simulink model "major"  (Simulink 7.4)
settings: Solver=ode23tb  StartTime=0.0  StopTime=2.5  RelTol=1e-3
InitFcn:
  | Ts=20e-6;
undefined symbols (not defined in the file): DiscIntNeverNeededParam, fc
libraries: powerlib x97, simulink x12, powerlib_extras x2
settings Model: Creator=srikanth  LastModifiedBy=Anil Pavuluru
settings DataIOCC: SaveOutput=off  SaveTime=off
settings DebuggingCC: AlgebraicLoopMsg=none

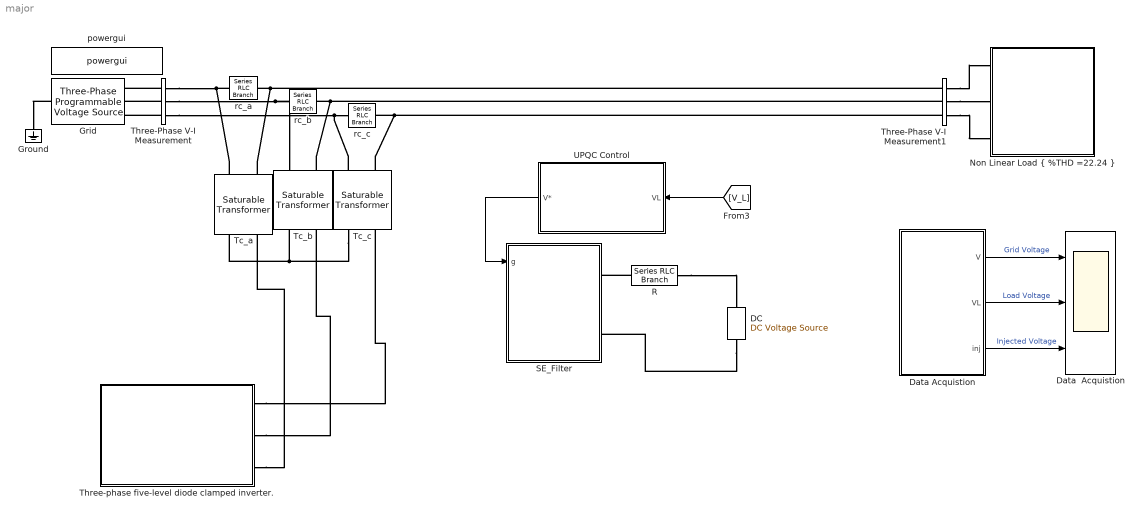
== system major ==
  DC : powerlib/Electrical Sources/DC Voltage Source  DialogController=POWERSYS.PowerSysDialog  SystemSampleTime=-1  Amplitude=700  Measurements=None
  Data  Acquistion : Scope  NumInputPorts=3
      settings: TickLabels=on  TimeRange=2.5  YMin=-350~-300~-200  YMax=350~350~225  SaveName=se_pi1
  Data Acquistion : Subsystem
      mask Display: fprintf('scopes')
  Grid : powerlib/Electrical Sources/Three-Phase Programmable Voltage Source  DialogController=POWERSYS.PowerSysDialog  SystemSampleTime=-1  PositiveSequence="[380  0 50]"  VariationEntity=Amplitude  VariationType=Table of time-amplitude pairs  VariationStep=0.5  VariationRate=10  VariationMagnitude=0.3  VariationFrequency=2  VariationTiming=[1 2]  VariationPhaseA=off  Amplitudes=[1 0.5 1 1.5 1]  TimeValues=[0 0.5 0.7 1.5 1.7]  HarmonicGeneration=on  HarmonicA=[5 0.2 0 2]  HarmonicB=[7 0.05 0 1]  Timing="[0.2  0.4]"
  Ground : powerlib/Elements/Ground  DialogController=POWERSYS.PowerSysDialog  PhysicalDomain=powersysdomain  SubClassName=unknown  LeftPortType=p1  RightPortType=p1  LConnTagsString=a
  "Non Linear Load { %THD =22.24 }" : Subsystem
      mask Display: fprintf('Non Linear\nLoad')
  R : powerlib/Elements/Series RLC Branch  DialogController=POWERSYS.PowerSysDialog  PhysicalDomain=powersysdomain  SubClassName=unknown  LeftPortType=p1  RightPortType=p1  LConnTagsString=__new0  RConnTagsString=__new0  BranchType=R  Resistance=0.1  Inductance=1e-3  SetiL0=off  InitialCurrent=0  Capacitance=1e-6  Setx0=off  InitialVoltage=0  Measurements=None
  SE_Filter : Subsystem
      mask Display: fprintf('series\nfilter')
  Tc_a : powerlib/Elements/Saturable Transformer  DialogController=POWERSYS.PowerSysDialog  SystemSampleTime=-1  ThreeWindings=off  UNITS=pu  NominalPower=[4000 50]  Winding1="[380  0.02  0.02 ]"  Winding2="[380  0.02  0.02]"  Winding3="[ 315e3  0.002  0.08 ]"  Saturation=[ 0 0 ;1.016 9.043]*1e-3  CoreLoss=[117 0]  Hysteresis=off  DataFile='hysteresis.mat'  Measurements=None  MoreParameters=off  BreakLoop=off  DataType=off  InitialFlux=0  TransfoNumber=1
  Tc_b : powerlib/Elements/Saturable Transformer  DialogController=POWERSYS.PowerSysDialog  SystemSampleTime=-1  ThreeWindings=off  UNITS=pu  NominalPower=[4000 50]  Winding1="[380  0.02  0.02 ]"  Winding2="[380  0.02  0.02]"  Winding3="[ 315e3  0.002  0.08 ]"  Saturation=[ 0 0 ;1.016 9.043]*1e-3  CoreLoss=[117 0]  Hysteresis=off  DataFile='hysteresis.mat'  Measurements=None  MoreParameters=off  BreakLoop=off  DataType=off  InitialFlux=0  TransfoNumber=1
  Tc_c : powerlib/Elements/Saturable Transformer  DialogController=POWERSYS.PowerSysDialog  SystemSampleTime=-1  ThreeWindings=off  UNITS=pu  NominalPower=[4000 50]  Winding1="[380  0.02  0.02 ]"  Winding2="[380  0.02  0.02]"  Winding3="[ 315e3  0.002  0.08 ]"  Saturation=[ 0 0 ;1.016 9.043]*1e-3  CoreLoss=[117 0]  Hysteresis=off  DataFile='hysteresis.mat'  Measurements=None  MoreParameters=off  BreakLoop=off  DataType=off  InitialFlux=0  TransfoNumber=1
  Three-Phase V-I Measurement : powerlib/Measurements/Three-Phase V-I Measurement  DialogController=POWERSYS.PowerSysDialog  SystemSampleTime=-1  VoltageMeasurement=phase-to-ground  SetLabelV=on  LabelV=Vabc  Vpu=off  CurrentMeasurement=yes  SetLabelI=on  LabelI=Iabc  Ipu=off  Pbase=100e6  Vbase=500e3  OutputType=Complex  PhasorSimulation=off  PSBequivalent=0
  Three-Phase V-I Measurement1 : powerlib/Measurements/Three-Phase V-I Measurement  DialogController=POWERSYS.PowerSysDialog  SystemSampleTime=-1  VoltageMeasurement=phase-to-ground  SetLabelV=on  LabelV=V_L  Vpu=off  CurrentMeasurement=yes  SetLabelI=on  LabelI=I_L  Ipu=off  Pbase=100e6  Vbase=500e3  OutputType=Complex  PhasorSimulation=off  PSBequivalent=0
  Three-phase five-level diode clamped inverter. : Subsystem
  UPQC Control : Subsystem
      mask Display: fprintf('Series\nFilter')
  powergui : powerlib/powergui  Priority=1  SystemSampleTime=-1  SimulationMode=Discrete  SampleTime=Ts  frequency=60  SPID=off  DisableSnubberDevices=off  DisableRonSwitches=off  DisableVfSwitches=off  SwTol=0  Interpol=off  frequencyindice=50  echomessages=off  HookPort=off  DisplayEquations=off  FunctionMessages=off  EnableUseOfTLC=off  x0status=blocks  RestoreLinks=warning  Frange=[0:2:500]  Ylog=off  Xlog=on  ShowGrid=off  save=off  variable=ZData  structure=voltage_pi  ZoomFFT=off  StartTime=1.5  cycles=10  DisplayStyle=1  fundamental=50  FreqAxis=on  MaxFrequency=1000  frequencyindicesteady=1  RmsSteady=1  display=off  Ts=0  methode=off
  rc_a : powerlib/Elements/Series RLC Branch  DialogController=POWERSYS.PowerSysDialog  PhysicalDomain=powersysdomain  SubClassName=unknown  LeftPortType=p1  RightPortType=p1  LConnTagsString=__new0  RConnTagsString=__new0  BranchType=RC  Resistance=1  Inductance=1e-3  SetiL0=off  InitialCurrent=0  Capacitance=100e-6  Setx0=off  InitialVoltage=0  Measurements=Branch voltage
  rc_b : powerlib/Elements/Series RLC Branch  DialogController=POWERSYS.PowerSysDialog  PhysicalDomain=powersysdomain  SubClassName=unknown  LeftPortType=p1  RightPortType=p1  LConnTagsString=__new0  RConnTagsString=__new0  BranchType=RC  Resistance=1  Inductance=1e-3  SetiL0=off  InitialCurrent=0  Capacitance=100e-6  Setx0=off  InitialVoltage=0  Measurements=Branch voltage
  rc_c : powerlib/Elements/Series RLC Branch  DialogController=POWERSYS.PowerSysDialog  PhysicalDomain=powersysdomain  SubClassName=unknown  LeftPortType=p1  RightPortType=p1  LConnTagsString=__new0  RConnTagsString=__new0  BranchType=RC  Resistance=1  Inductance=1e-3  SetiL0=off  InitialCurrent=0  Capacitance=100e-6  Setx0=off  InitialVoltage=0  Measurements=Branch voltage
  wires:
  [V_L] -> UPQC Control/1(VL)
  UPQC Control/1(V*) -> SE_Filter/1(g)
  Data Acquistion/1(V) -> Data  Acquistion/1  "Grid Voltage"
  Data Acquistion/2(VL) -> Data  Acquistion/2  "Load Voltage"
  Data Acquistion/3("inj ") -> Data  Acquistion/3  "Injected Voltage"
  connections:
  Three-Phase V-I Measurement1/LConn2 -- rc_b/LConn1 -- Tc_b/RConn2
  Three-Phase V-I Measurement1/LConn1 -- rc_a/LConn1 -- Tc_a/RConn2
  Grid/LConn1 -- Ground/LConn1
  Three-Phase V-I Measurement/LConn1 -- Grid/RConn1
  Three-Phase V-I Measurement/LConn2 -- Grid/RConn2
  Three-Phase V-I Measurement/LConn3 -- Grid/RConn3
  Three-Phase V-I Measurement1/RConn2 -- "Non Linear Load { %THD =22.24 }"/LConn2
  Three-Phase V-I Measurement1/LConn3 -- rc_c/LConn1 -- Tc_c/RConn2
  rc_a/RConn1 -- Three-Phase V-I Measurement/RConn1 -- Tc_a/RConn1
  rc_b/RConn1 -- Three-Phase V-I Measurement/RConn2 -- Tc_b/RConn1
  rc_c/RConn1 -- Three-Phase V-I Measurement/RConn3 -- Tc_c/RConn1
  Three-Phase V-I Measurement1/RConn3 -- "Non Linear Load { %THD =22.24 }"/LConn3
  Three-Phase V-I Measurement1/RConn1 -- "Non Linear Load { %THD =22.24 }"/LConn1
  Three-phase five-level diode clamped inverter./RConn3 -- Tc_a/LConn2
  Three-phase five-level diode clamped inverter./RConn2 -- Tc_b/LConn2
  Three-phase five-level diode clamped inverter./RConn1 -- Tc_c/LConn2
  Tc_c/LConn1 -- Tc_a/LConn1 -- Tc_b/LConn1
  R/LConn1 -- SE_Filter/RConn1
  R/RConn1 -- DC/RConn1
  DC/LConn1 -- SE_Filter/RConn2

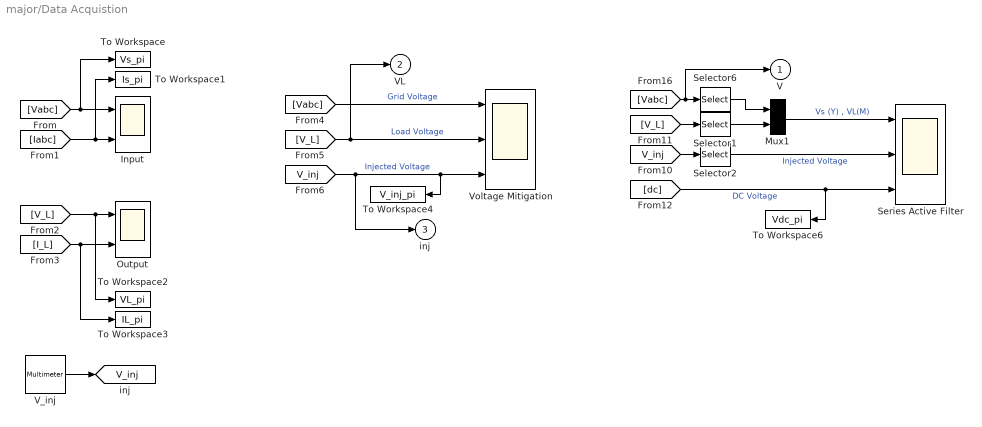
== system major/Data Acquistion ==
  Input : Scope  NumInputPorts=2
      settings: TimeRange=0.1  YMin=-400~-15  YMax=400~15  SaveName=Grid_pi
  Mux1 : Mux  Inputs=2
      settings: DisplayOption=signals
  Output : Scope  NumInputPorts=2
      settings: TimeRange=0.1  YMin=-400~-10  YMax=400~10  SaveName=Load_pi
  Selector1 : Selector  InputPortWidth=3  IndexOptions=Index vector (dialog)  Indices=1  OutputSizes=1
  Selector2 : Selector  InputPortWidth=3  IndexOptions=Index vector (dialog)  Indices=1  OutputSizes=1
  Selector6 : Selector  InputPortWidth=3  IndexOptions=Index vector (dialog)  Indices=1  OutputSizes=1
  Series Active Filter : Scope  NumInputPorts=3
      settings: TickLabels=on  TimeRange=2  YMin=-350~-175~600  YMax=350~175~1000  SaveName=se_pi
  To Workspace : ToWorkspace  VariableName=Vs_pi  SampleTime=Ts  SaveFormat=Array
  To Workspace1 : ToWorkspace  VariableName=Is_pi  SampleTime=Ts  SaveFormat=Array
  To Workspace2 : ToWorkspace  VariableName=VL_pi  SampleTime=Ts  SaveFormat=Array
  To Workspace3 : ToWorkspace  VariableName=IL_pi  SampleTime=Ts  SaveFormat=Array
  To Workspace4 : ToWorkspace  VariableName=V_inj_pi  SampleTime=Ts  SaveFormat=Array
  To Workspace6 : ToWorkspace  VariableName=Vdc_pi  SampleTime=Ts  SaveFormat=Array
  V_inj : powerlib/Measurements/Multimeter  SystemSampleTime=-1  PhasorSimulation=off  OutputType=Complex  sel=[1 2 3]  L=7  Gain=[1 1 1]  yselected={'Ub: rc_a','Ub: rc_b','Ub: rc_c'};  PSBOutputType=1  PSBequivalent=0  AxesSetting=[0,0.1,-100,100]  Display=0  SavedBlockNames=-11
  Voltage Mitigation : Scope  NumInputPorts=3
      settings: TimeRange=0.2  YMin=-500~-500~-200  YMax=500~500~200  SaveName=voltage_pi
  V : Outport  OutDataType=fixdt(1, 16)  OutScaling=2^0
  VL : Outport  Port=2  OutDataType=fixdt(1, 16)  OutScaling=2^0
  "inj " : Outport  Port=3  OutDataType=fixdt(1, 16)  OutScaling=2^0
  tag scope: V_inj=global
  wires:
  [Vabc] -> Input/1, To Workspace/1
  [Iabc] -> Input/2, To Workspace1/1
  [V_L] -> Output/1, To Workspace2/1
  [I_L] -> Output/2, To Workspace3/1
  [Vabc] -> Voltage Mitigation/1  "Grid Voltage"
  [V_L] -> Voltage Mitigation/2, VL/1  "Load Voltage"
  [V_inj] -> Voltage Mitigation/3, To Workspace4/1, "inj "/1  "Injected Voltage"
  [V_L] -> Selector1/1
  [V_inj] -> Selector2/1
  [dc] -> Series Active Filter/3, To Workspace6/1  "DC Voltage"
  Selector2/1 -> Series Active Filter/2  "Injected Voltage"
  [Vabc] -> Selector6/1, V/1
  Selector1/1 -> Mux1/2
  Mux1/1 -> Series Active Filter/1  "Vs (Y) , VL(M)"
  Selector6/1 -> Mux1/1
  V_inj/1 -> [V_inj]

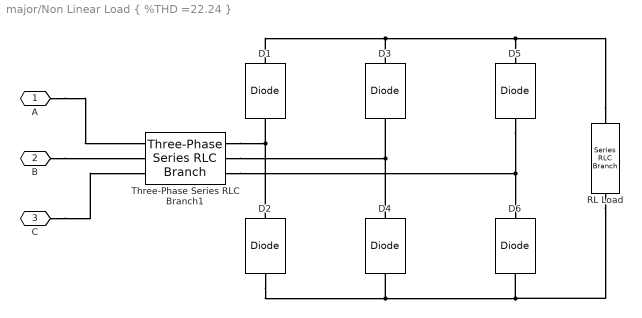
== system major/Non Linear Load { %THD =22.24 } ==
  D{1..6} (6 alike) : powerlib/Power Electronics/Diode  DialogController=POWERSYS.PowerSysDialog  SystemSampleTime=-1  Ron=0.001  Lon=0  Vf=0.8  IC=0  UseSnubber=off  Rs=500  Cs=250e-9  Measurements=off
  RL Load : powerlib/Elements/Series RLC Branch  DialogController=POWERSYS.PowerSysDialog  PhysicalDomain=powersysdomain  SubClassName=unknown  LeftPortType=p1  RightPortType=p1  LConnTagsString=__new0  RConnTagsString=__new0  BranchType=RL  Resistance=60  Inductance=0.15e-3  SetiL0=off  InitialCurrent=0  Capacitance=1e-6  Setx0=off  InitialVoltage=0  Measurements=None
  Three-Phase Series RLC Branch1 : powerlib/Elements/Three-Phase Series RLC Branch  DialogController=POWERSYS.PowerSysDialog  PhysicalDomain=powersysdomain  SubClassName=unknown  LeftPortType=p1  RightPortType=p1  LConnTagsString=A|B|C  RConnTagsString=A|B|C  BranchType=RL  Resistance=0.4  Inductance=15e-3  Capacitance=1e-6  Measurements=None
  A : PMIOPort  Port=1  Side=Left
  B : PMIOPort  Port=2  Side=Left
  C : PMIOPort  Port=3  Side=Left
  connections:
  C/RConn1 -- Three-Phase Series RLC Branch1/LConn3
  B/RConn1 -- Three-Phase Series RLC Branch1/LConn2
  A/RConn1 -- Three-Phase Series RLC Branch1/LConn1
  Three-Phase Series RLC Branch1/RConn3 -- D6/RConn1 -- D5/LConn1
  Three-Phase Series RLC Branch1/RConn2 -- D4/RConn1 -- D3/LConn1
  RL Load/RConn1 -- D6/LConn1 -- D4/LConn1 -- D2/LConn1
  RL Load/LConn1 -- D5/RConn1 -- D3/RConn1 -- D1/RConn1
  Three-Phase Series RLC Branch1/RConn1 -- D2/RConn1 -- D1/LConn1

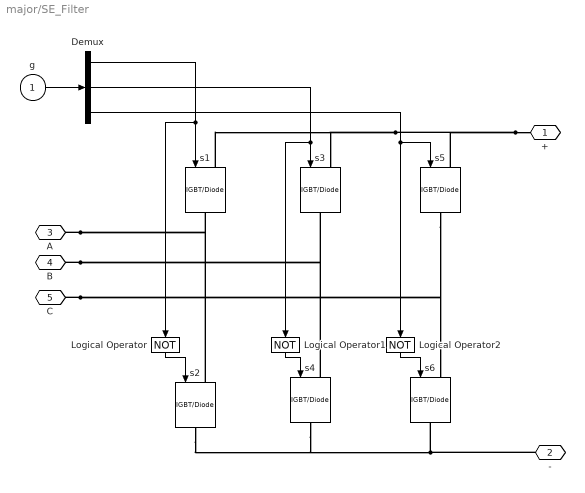
== system major/SE_Filter ==
  g : Inport
  Demux : Demux  Outputs=3
  Logical Operator : Logic  Operator=NOT  AllPortsSameDT=off  OutDataTypeMode=boolean  LogicDataType=fixdt(0, 8)  OutDataTypeStr=boolean
  Logical Operator1 : Logic  Operator=NOT  AllPortsSameDT=off  OutDataTypeMode=boolean  LogicDataType=fixdt(0, 8)  OutDataTypeStr=boolean
  Logical Operator2 : Logic  Operator=NOT  AllPortsSameDT=off  OutDataTypeMode=boolean  LogicDataType=fixdt(0, 8)  OutDataTypeStr=boolean
  s{1..6} (6 alike) : powerlib/Power Electronics/IGBT//Diode  DialogController=POWERSYS.PowerSysDialog  SystemSampleTime=-1  Ron=1e-3  Rs=1e5  Cs=inf  Measurements=off
  + : PMIOPort  Port=1  Side=Right
  - : PMIOPort  Port=2  Side=Right
  A : PMIOPort  Port=3  Side=Left
  B : PMIOPort  Port=4  Side=Left
  C : PMIOPort  Port=5  Side=Left
  wires:
  Demux/2 -> s3/1, Logical Operator1/1
  Demux/1 -> s1/1, Logical Operator/1
  Logical Operator/1 -> s2/1
  Logical Operator1/1 -> s4/1
  Logical Operator2/1 -> s6/1
  Demux/3 -> Logical Operator2/1, s5/1
  g/1 -> Demux/1
  connections:
  +/RConn1 -- s5/LConn1 -- s1/LConn1 -- s3/LConn1
  A/RConn1 -- s2/LConn1 -- s1/RConn1
  -/RConn1 -- s6/RConn1 -- s4/RConn1 -- s2/RConn1
  B/RConn1 -- s4/LConn1 -- s3/RConn1
  C/RConn1 -- s5/RConn1 -- s6/LConn1

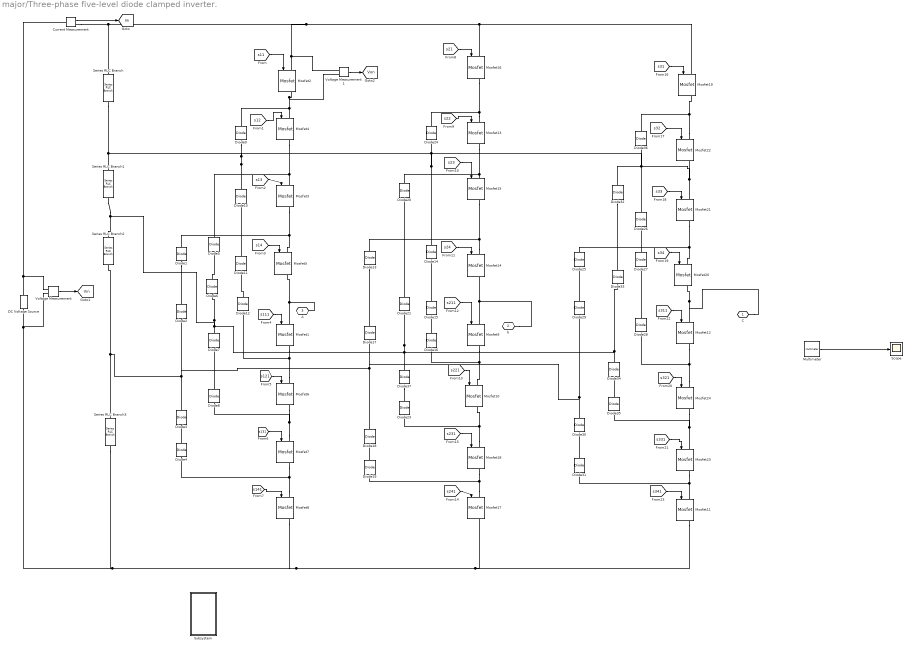
== system major/Three-phase five-level diode clamped inverter. ==
  Current Measurement : powerlib/Measurements/Current Measurement  DialogController=POWERSYS.PowerSysDialog  SystemSampleTime=-1  PhasorSimulation=off  OutputType=Complex  PSBequivalent=0
  DC Voltage Source : powerlib/Electrical Sources/DC Voltage Source  DialogController=POWERSYS.PowerSysDialog  SystemSampleTime=-1  Amplitude=500  Measurements=None
  Diode{1..21,23..37} (36 alike) : powerlib/Power Electronics/Diode  DialogController=POWERSYS.PowerSysDialog  SystemSampleTime=-1  Ron=0.001  Lon=0  Vf=0.8  IC=0  UseSnubber=off  Rs=500  Cs=250e-9  Measurements=off
  Mosfet{1..24} (24 alike) : powerlib/Power Electronics/Mosfet  DialogController=POWERSYS.PowerSysDialog  SystemSampleTime=-1  Ron=0.1  Lon=0  Rd=0.01  Vfd=0  IC=0  Rs=1e5  Cs=inf  Measurements=on
  Multimeter : powerlib/Measurements/Multimeter  SystemSampleTime=-1  PhasorSimulation=off  OutputType=Complex  sel=[4 5 6 7]  L=7  Gain=[1 1 1 1]  yselected={'Ub: Three-phase five-level diode clamped inverter./Series RLC Branch','Ub: Three-phase five-level diode clamped inverter./Series RLC Branch1','Ub: Three-phase five-level diode clamped inverter./Series RLC Branch2','Ub: Three-phase five-level diode clamped inverter./Series RLC Branch3'};  PSBOutputType=1  PSBequivalent=0  AxesSetting=[0,0.1,-100,100]  Display=0  SavedBlockNames=-11
  Scope : Scope
      settings: YMin=-150  YMax=150  SaveName=ScopeData4
  Series RLC Branch{,1..3} (4 alike) : powerlib/Elements/Series RLC Branch  DialogController=POWERSYS.PowerSysDialog  PhysicalDomain=powersysdomain  SubClassName=unknown  LeftPortType=p1  RightPortType=p1  LConnTagsString=__new0  RConnTagsString=__new0  BranchType=RC  Resistance=0.01  Inductance=1e-3  SetiL0=off  InitialCurrent=0  Capacitance=200e-3  Setx0=off  InitialVoltage=0  Measurements=Branch voltage
  Subsystem : Subsystem
  Voltage Measurement : powerlib/Measurements/Voltage Measurement  DialogController=POWERSYS.PowerSysDialog  SystemSampleTime=-1  PhasorSimulation=off  OutputType=Complex  PSBequivalent=0
  Voltage Measurement1 : powerlib/Measurements/Voltage Measurement  DialogController=POWERSYS.PowerSysDialog  SystemSampleTime=-1  PhasorSimulation=off  OutputType=Complex  PSBequivalent=0
  C : PMIOPort  Tag=PMCPort  Port=1  Side=Right
  b : PMIOPort  Tag=PMCPort  Port=2  Side=Right
  A : PMIOPort  Tag=PMCPort  Port=3  Side=Right
  tag scope: Iin=global, Vin=global, Von=global
  wires:
  [s141] -> Mosfet8/1
  [s131] -> Mosfet7/1
  [s121] -> Mosfet6/1
  [s111] -> Mosfet1/1
  [s14] -> Mosfet5/1
  [s13] -> Mosfet3/1
  [s12] -> Mosfet4/1
  [s11] -> Mosfet2/1
  [s241] -> Mosfet17/1
  [s231] -> Mosfet18/1
  [s221] -> Mosfet10/1
  [s211] -> Mosfet9/1
  [s24] -> Mosfet14/1
  [s23] -> Mosfet15/1
  [s22] -> Mosfet13/1
  [s21] -> Mosfet16/1
  [s341] -> Mosfet11/1
  [s331] -> Mosfet23/1
  [s321] -> Mosfet24/1
  [s311] -> Mosfet12/1
  [s34] -> Mosfet20/1
  [s33] -> Mosfet21/1
  [s32] -> Mosfet22/1
  [s31] -> Mosfet19/1
  Multimeter/1 -> Scope/1
  Current Measurement/1 -> [Iin]
  Voltage Measurement/1 -> [Vin]
  Voltage Measurement1/1 -> [Von]
  connections:
  Series RLC Branch3/LConn1 -- Mosfet17/RConn1 -- Mosfet11/RConn1 -- Mosfet8/RConn1 -- DC Voltage Source/LConn1 -- Voltage Measurement/LConn2
  Mosfet16/LConn1 -- Mosfet19/LConn1 -- Series RLC Branch/LConn1 -- Current Measurement/RConn1 -- Mosfet2/LConn1 -- Voltage Measurement1/LConn1
  Series RLC Branch3/RConn1 -- Diode3/RConn1 -- Diode2/LConn1 -- Diode18/RConn1 -- Diode17/LConn1 -- Diode30/RConn1 -- Diode29/LConn1 -- Series RLC Branch2/LConn1
  Mosfet5/LConn1 -- Diode1/RConn1 -- Mosfet3/RConn1
  Diode11/RConn1 -- Diode10/LConn1
  Series RLC Branch1/LConn1 -- Diode10/RConn1 -- Diode9/LConn1 -- Diode14/RConn1 -- Diode24/LConn1 -- Diode26/RConn1 -- Diode36/LConn1 -- Series RLC Branch/RConn1
  Diode12/RConn1 -- Diode11/LConn1
  Mosfet6/LConn1 -- Diode12/LConn1 -- Mosfet1/RConn1
  Mosfet14/LConn1 -- Diode13/RConn1 -- Mosfet15/RConn1
  Diode15/RConn1 -- Diode14/LConn1
  Diode16/RConn1 -- Diode15/LConn1
  Mosfet10/LConn1 -- Diode16/LConn1 -- Mosfet9/RConn1
  Diode19/RConn1 -- Diode18/LConn1
  Mosfet17/LConn1 -- Diode19/LConn1 -- Mosfet18/RConn1
  Diode21/RConn1 -- Diode20/LConn1
  Diode37/LConn1 -- Diode23/RConn1
  Mosfet18/LConn1 -- Diode23/LConn1 -- Mosfet10/RConn1
  Mosfet13/LConn1 -- Diode24/RConn1 -- Mosfet16/RConn1
  Mosfet20/LConn1 -- Diode25/RConn1 -- Mosfet21/RConn1
  Diode27/RConn1 -- Diode26/LConn1
  Diode28/RConn1 -- Diode27/LConn1
  Mosfet24/LConn1 -- Diode28/LConn1 -- Mosfet12/RConn1
  Diode4/RConn1 -- Diode3/LConn1
  Diode31/RConn1 -- Diode30/LConn1
  Mosfet23/RConn1 -- Diode31/LConn1 -- Mosfet11/LConn1
  Mosfet21/LConn1 -- Diode32/RConn1 -- Mosfet22/RConn1
  Series RLC Branch2/RConn1 -- Diode34/RConn1 -- Diode33/LConn1 -- Diode37/RConn1 -- Diode21/LConn1 -- Diode7/RConn1 -- Diode6/LConn1 -- Series RLC Branch1/RConn1
  Diode35/RConn1 -- Diode34/LConn1
  Mosfet24/RConn1 -- Diode35/LConn1 -- Mosfet23/LConn1
  Mosfet22/LConn1 -- Diode36/RConn1 -- Mosfet19/RConn1
  Mosfet8/LConn1 -- Diode4/LConn1 -- Mosfet7/RConn1
  Diode6/RConn1 -- Diode5/LConn1
  Diode8/RConn1 -- Diode7/LConn1
  Mosfet7/LConn1 -- Diode8/LConn1 -- Mosfet6/RConn1
  Mosfet2/RConn1 -- Mosfet4/LConn1 -- Diode9/RConn1 -- Voltage Measurement1/LConn2
  Mosfet9/LConn1 -- b/RConn1 -- Mosfet14/RConn1
  Mosfet1/LConn1 -- A/RConn1 -- Mosfet5/RConn1
  Mosfet12/LConn1 -- C/RConn1 -- Mosfet20/RConn1
  Diode29/RConn1 -- Diode25/LConn1
  Diode1/LConn1 -- Diode2/RConn1
  Diode32/LConn1 -- Diode33/RConn1
  Diode5/RConn1 -- Mosfet3/LConn1 -- Mosfet4/RConn1
  Mosfet13/RConn1 -- Mosfet15/LConn1 -- Diode20/RConn1
  Diode13/LConn1 -- Diode17/RConn1
  DC Voltage Source/RConn1 -- Current Measurement/LConn1 -- Voltage Measurement/LConn1

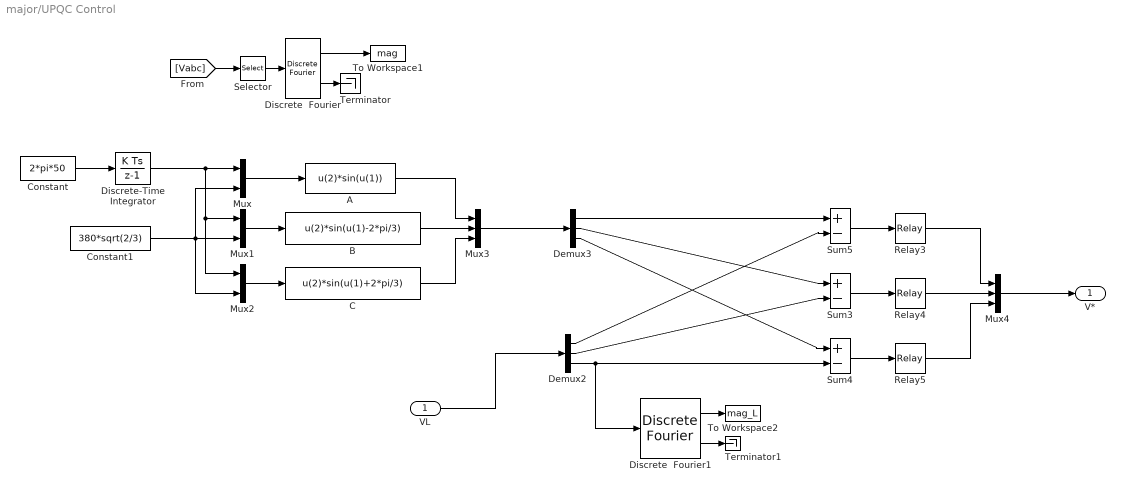
== system major/UPQC Control ==
  VL : Inport
  A : Fcn  Expr=u(2)*sin(u(1))
  B : Fcn  Expr=u(2)*sin(u(1)-2*pi/3)
  C : Fcn  Expr=u(2)*sin(u(1)+2*pi/3)
  Constant : Constant  Value=2*pi*50  OutDataType=fixdt(1, 16)  OutScaling=2^0
  Constant1 : Constant  Value=380*sqrt(2/3)  OutDataType=fixdt(1, 16)  OutScaling=2^0
  Demux2 : Demux  Outputs=3
  Demux3 : Demux  Outputs=3
  Discrete  Fourier : powerlib_extras/Discrete Measurements/Discrete  Fourier  DialogController=POWERSYS.PowerSysDialog  SystemSampleTime=-1  Freq=50  n=1  Par_Init=[0 0]  Ts=Ts
  Discrete  Fourier1 : powerlib_extras/Discrete Measurements/Discrete  Fourier  DialogController=POWERSYS.PowerSysDialog  SystemSampleTime=-1  Freq=50  n=1  Par_Init=[0 0]  Ts=Ts
  Discrete-Time Integrator : DiscreteIntegrator  SampleTime=Ts  OutDataType=fixdt(1, 16)  OutScaling=2^0  ICPrevOutput=DiscIntNeverNeededParam  ICPrevScaledInput=DiscIntNeverNeededParam
  Mux : Mux  Inputs=2
  Mux1 : Mux  Inputs=2
  Mux2 : Mux  Inputs=2
  Mux3 : Mux  Inputs=3
  Mux4 : Mux  Inputs=3
  Relay3 : Relay  OnSwitchValue=1  OffSwitchValue=-1  OutDataType=fixdt(1, 16)  OutScaling=2^0
  Relay4 : Relay  OnSwitchValue=1  OffSwitchValue=-1  OutDataType=fixdt(1, 16)  OutScaling=2^0
  Relay5 : Relay  OnSwitchValue=1  OffSwitchValue=-1  OutDataType=fixdt(1, 16)  OutScaling=2^0
  Selector : Selector  InputPortWidth=3  IndexOptions=Index vector (dialog)  Indices=1  OutputSizes=1
  Sum3 : Sum  Inputs=+-  OutDataType=fixdt(1, 16)  OutScaling=2^0
  Sum4 : Sum  Inputs=+-  OutDataType=fixdt(1, 16)  OutScaling=2^0
  Sum5 : Sum  Inputs=+-  OutDataType=fixdt(1, 16)  OutScaling=2^0
  Terminator : Terminator
  Terminator1 : Terminator
  To Workspace1 : ToWorkspace  VariableName=mag  SampleTime=Ts  SaveFormat=Array
  To Workspace2 : ToWorkspace  VariableName=mag_L  SampleTime=Ts  SaveFormat=Array
  V* : Outport  OutDataType=fixdt(1, 16)  OutScaling=2^0
  wires:
  Constant/1 -> Discrete-Time Integrator/1
  Discrete-Time Integrator/1 -> Mux/1, Mux2/1, Mux1/1
  Constant1/1 -> Mux/2, Mux1/2, Mux2/2
  Mux/1 -> A/1
  Mux1/1 -> B/1
  Mux2/1 -> C/1
  Discrete  Fourier/2 -> Terminator/1
  Selector/1 -> Discrete  Fourier/1
  [Vabc] -> Selector/1
  Discrete  Fourier/1 -> To Workspace1/1
  A/1 -> Mux3/1
  B/1 -> Mux3/2
  C/1 -> Mux3/3
  Discrete  Fourier1/2 -> Terminator1/1
  Sum5/1 -> Relay3/1
  Sum3/1 -> Relay4/1
  Sum4/1 -> Relay5/1
  Relay3/1 -> Mux4/1
  Relay4/1 -> Mux4/2
  Relay5/1 -> Mux4/3
  Mux4/1 -> V*/1
  Discrete  Fourier1/1 -> To Workspace2/1
  VL/1 -> Demux2/1
  Demux3/1 -> Sum5/1
  Demux2/3 -> Sum4/2, Discrete  Fourier1/1
  Demux2/1 -> Sum5/2
  Demux3/3 -> Sum4/1
  Demux2/2 -> Sum3/2
  Demux3/2 -> Sum3/1
  Mux3/1 -> Demux3/1

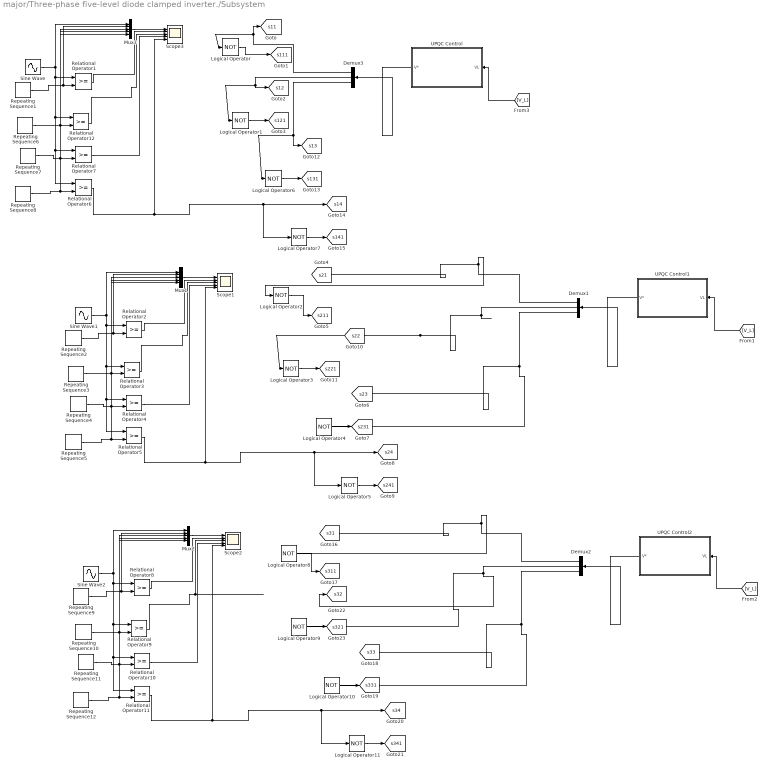
== system major/Three-phase five-level diode clamped inverter./Subsystem ==
  Demux1 : Demux  Outputs=3
  Demux2 : Demux  Outputs=3
  Demux3 : Demux  Outputs=3
  Logical Operator{,1..11} (12 alike) : Logic  Operator=NOT  AllPortsSameDT=off  OutDataTypeMode=boolean  OutDataTypeStr=boolean
  Mux1 : Mux  Inputs=5
  Mux2 : Mux  Inputs=5
  Mux3 : Mux  Inputs=5
  Relational Operator{1..12} (12 alike) : RelationalOperator  LogicOutDataTypeMode=boolean  OutDataTypeStr=boolean
  Repeating Sequence1 : simulink/Sources/Repeating Sequence  SystemSampleTime=-1  rep_seq_t=[0 1/fc/4 3/fc/4 1/fc]  rep_seq_y="[1.5  2 1 1.5]"
  Repeating Sequence10 : simulink/Sources/Repeating Sequence  SystemSampleTime=-1  rep_seq_t=[0 1/fc/4 3/fc/4 1/fc]  rep_seq_y=[0.5 1 0 0.5]
  Repeating Sequence11 : simulink/Sources/Repeating Sequence  SystemSampleTime=-1  rep_seq_t=[0 1/fc/4 3/fc/4 1/fc]  rep_seq_y=[-0.5 0 -1 -0.5]
  Repeating Sequence12 : simulink/Sources/Repeating Sequence  SystemSampleTime=-1  rep_seq_t=[0 1/fc/4 3/fc/4 1/fc]  rep_seq_y="[-1.5  -1 -2 -1.5]"
  Repeating Sequence2 : simulink/Sources/Repeating Sequence  SystemSampleTime=-1  rep_seq_t=[0 1/fc/4 3/fc/4 1/fc]  rep_seq_y="[1.5  2 1 1.5]"
  Repeating Sequence3 : simulink/Sources/Repeating Sequence  SystemSampleTime=-1  rep_seq_t=[0 1/fc/4 3/fc/4 1/fc]  rep_seq_y=[0.5 1 0 0.5]
  Repeating Sequence4 : simulink/Sources/Repeating Sequence  SystemSampleTime=-1  rep_seq_t=[0 1/fc/4 3/fc/4 1/fc]  rep_seq_y=[-0.5 0 -1 -0.5]
  Repeating Sequence5 : simulink/Sources/Repeating Sequence  SystemSampleTime=-1  rep_seq_t=[0 1/fc/4 3/fc/4 1/fc]  rep_seq_y="[-1.5  -1 -2 -1.5]"
  Repeating Sequence6 : simulink/Sources/Repeating Sequence  SystemSampleTime=-1  rep_seq_t=[0 1/fc/4 3/fc/4 1/fc]  rep_seq_y=[0.5 1 0 0.5]
  Repeating Sequence7 : simulink/Sources/Repeating Sequence  SystemSampleTime=-1  rep_seq_t=[0 1/fc/4 3/fc/4 1/fc]  rep_seq_y=[-0.5 0 -1 -0.5]
  Repeating Sequence8 : simulink/Sources/Repeating Sequence  SystemSampleTime=-1  rep_seq_t=[0 1/fc/4 3/fc/4 1/fc]  rep_seq_y="[-1.5  -1 -2 -1.5]"
  Repeating Sequence9 : simulink/Sources/Repeating Sequence  SystemSampleTime=-1  rep_seq_t=[0 1/fc/4 3/fc/4 1/fc]  rep_seq_y="[1.5  2 1 1.5]"
  Scope1 : Scope  NumInputPorts=5
      settings: TimeRange=10  YMin=-3~0~0~-5~-5  YMax=3~1~1~5~5
  Scope2 : Scope  NumInputPorts=5
      settings: TimeRange=0.5  YMin=-2~0~0~0~0  YMax=2~1~1~1~1  SaveName=ScopeData2
  Scope3 : Scope  NumInputPorts=5
      settings: TimeRange=0.06  YMin=-2~-1~0~0~0.95  YMax=2~1~1~1~1.05
  Sine Wave : Sin  Amplitude=2  Bias=0  Frequency=2*pi*50  Phase=0  Samples=10  SampleTime=50e-6  Offset=0
  Sine Wave1 : Sin  Amplitude=2  Bias=0  Frequency=2*pi*50  Phase=2*pi/3  Samples=10  SampleTime=50e-6  Offset=0
  Sine Wave2 : Sin  Amplitude=2  Bias=0  Frequency=2*pi*50  Phase=-2*pi/3  Samples=10  SampleTime=50e-6  Offset=0
  UPQC Control : Subsystem
      mask Display: fprintf('Series\nFilter')
  UPQC Control1 : Subsystem
      mask Display: fprintf('Series\nFilter')
  UPQC Control2 : Subsystem
      mask Display: fprintf('Series\nFilter')
  tag scope: s111=global, s11=global, s121=global, s12=global, s131=global, s13=global, s141=global, s14=global, s211=global, s21=global, s221=global, s22=global, s231=global, s23=global, s241=global, s24=global, s311=global, s31=global, s321=global, s32=global, s331=global, s33=global, s341=global, s34=global
  wires:
  Sine Wave/1 -> Relational Operator6/1, Relational Operator7/1, Relational Operator12/1, Relational Operator1/1, Mux3/1
  Repeating Sequence1/1 -> Mux3/2, Relational Operator1/2
  Repeating Sequence6/1 -> Mux3/3, Relational Operator12/2
  Relational Operator1/1 -> Scope3/2
  Relational Operator12/1 -> Scope3/3
  Logical Operator/1 -> [s111]
  Logical Operator1/1 -> [s121]
  Repeating Sequence7/1 -> Mux3/4, Relational Operator7/2
  Repeating Sequence8/1 -> Mux3/5, Relational Operator6/2
  Relational Operator7/1 -> Scope3/4
  Logical Operator6/1 -> [s131]
  Relational Operator6/1 -> [s14], Logical Operator7/1, Scope3/5
  Logical Operator7/1 -> [s141]
  Mux3/1 -> Scope3/1
  Sine Wave1/1 -> Relational Operator5/1, Relational Operator4/1, Relational Operator3/1, Relational Operator2/1, Mux1/1
  Repeating Sequence2/1 -> Mux1/2, Relational Operator2/2
  Repeating Sequence3/1 -> Mux1/3, Relational Operator3/2
  Relational Operator2/1 -> Scope1/2
  Relational Operator3/1 -> Scope1/3
  Logical Operator2/1 -> [s211]
  Logical Operator3/1 -> [s221]
  Repeating Sequence4/1 -> Mux1/4, Relational Operator4/2
  Repeating Sequence5/1 -> Mux1/5, Relational Operator5/2
  Relational Operator4/1 -> Scope1/4
  Logical Operator4/1 -> [s231]
  Relational Operator5/1 -> [s24], Logical Operator5/1, Scope1/5
  Logical Operator5/1 -> [s241]
  Mux1/1 -> Scope1/1
  Sine Wave2/1 -> Relational Operator11/1, Relational Operator10/1, Relational Operator9/1, Relational Operator8/1, Mux2/1
  Repeating Sequence9/1 -> Mux2/2, Relational Operator8/2
  Repeating Sequence10/1 -> Mux2/3, Relational Operator9/2
  Relational Operator8/1 -> Scope2/2
  Relational Operator9/1 -> Scope2/3
  Logical Operator8/1 -> [s311]
  Logical Operator9/1 -> [s321]
  Repeating Sequence11/1 -> Mux2/4, Relational Operator10/2
  Repeating Sequence12/1 -> Mux2/5, Relational Operator11/2
  Relational Operator10/1 -> Scope2/4
  Logical Operator10/1 -> [s331]
  Relational Operator11/1 -> [s34], Logical Operator11/1, Scope2/5
  Logical Operator11/1 -> [s341]
  Mux2/1 -> Scope2/1
  [V_L] -> UPQC Control/1(VL)
  UPQC Control/1(V*) -> Demux3/1
  Demux3/1 -> [s11], Logical Operator/1
  Demux3/2 -> [s12], Logical Operator1/1
  Demux3/3 -> [s13], Logical Operator6/1
  [V_L] -> UPQC Control1/1(VL)
  UPQC Control1/1(V*) -> Demux1/1
  Demux1/1 -> [s21], Logical Operator2/1
  Demux1/2 -> [s22], Logical Operator3/1
  Demux1/3 -> [s23], Logical Operator4/1
  [V_L] -> UPQC Control2/1(VL)
  UPQC Control2/1(V*) -> Demux2/1
  Demux2/1 -> [s31], Logical Operator8/1
  Demux2/2 -> [s32], Logical Operator9/1
  Demux2/3 -> [s33], Logical Operator10/1

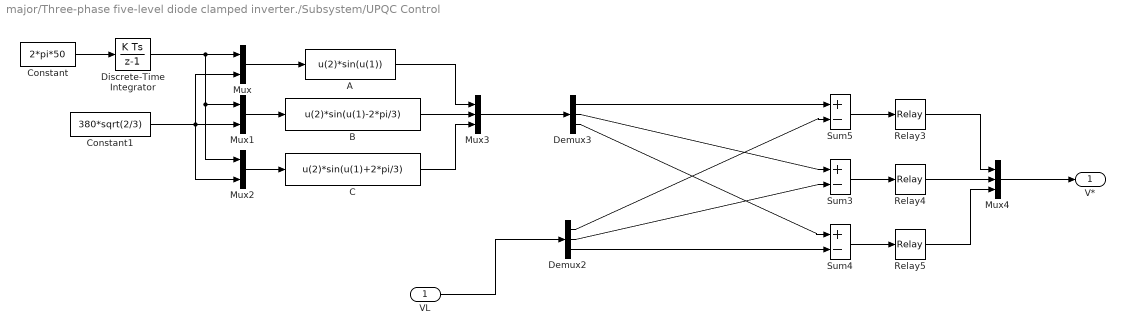
== system major/Three-phase five-level diode clamped inverter./Subsystem/UPQC Control ==
  VL : Inport
  A : Fcn  Expr=u(2)*sin(u(1))
  B : Fcn  Expr=u(2)*sin(u(1)-2*pi/3)
  C : Fcn  Expr=u(2)*sin(u(1)+2*pi/3)
  Constant : Constant  Value=2*pi*50  OutDataType=fixdt(1, 16)  OutScaling=2^0
  Constant1 : Constant  Value=380*sqrt(2/3)  OutDataType=fixdt(1, 16)  OutScaling=2^0
  Demux2 : Demux  Outputs=3
  Demux3 : Demux  Outputs=3
  Discrete-Time Integrator : DiscreteIntegrator  SampleTime=Ts  OutDataType=fixdt(1, 16)  OutScaling=2^0  ICPrevOutput=DiscIntNeverNeededParam  ICPrevScaledInput=DiscIntNeverNeededParam
  Mux : Mux  Inputs=2
  Mux1 : Mux  Inputs=2
  Mux2 : Mux  Inputs=2
  Mux3 : Mux  Inputs=3
  Mux4 : Mux  Inputs=3
  Relay3 : Relay  OnSwitchValue=1  OffSwitchValue=-1  OutDataType=fixdt(1, 16)  OutScaling=2^0
  Relay4 : Relay  OnSwitchValue=1  OffSwitchValue=-1  OutDataType=fixdt(1, 16)  OutScaling=2^0
  Relay5 : Relay  OnSwitchValue=1  OffSwitchValue=-1  OutDataType=fixdt(1, 16)  OutScaling=2^0
  Sum3 : Sum  Inputs=+-  OutDataType=fixdt(1, 16)  OutScaling=2^0
  Sum4 : Sum  Inputs=+-  OutDataType=fixdt(1, 16)  OutScaling=2^0
  Sum5 : Sum  Inputs=+-  OutDataType=fixdt(1, 16)  OutScaling=2^0
  V* : Outport  OutDataType=fixdt(1, 16)  OutScaling=2^0
  wires:
  Constant/1 -> Discrete-Time Integrator/1
  Discrete-Time Integrator/1 -> Mux/1, Mux2/1, Mux1/1
  Constant1/1 -> Mux/2, Mux1/2, Mux2/2
  Mux/1 -> A/1
  Mux1/1 -> B/1
  Mux2/1 -> C/1
  A/1 -> Mux3/1
  B/1 -> Mux3/2
  C/1 -> Mux3/3
  Sum5/1 -> Relay3/1
  Sum3/1 -> Relay4/1
  Sum4/1 -> Relay5/1
  Relay3/1 -> Mux4/1
  Relay4/1 -> Mux4/2
  Relay5/1 -> Mux4/3
  Mux4/1 -> V*/1
  VL/1 -> Demux2/1
  Demux3/1 -> Sum5/1
  Demux2/3 -> Sum4/2
  Demux2/1 -> Sum5/2
  Demux3/3 -> Sum4/1
  Demux2/2 -> Sum3/2
  Demux3/2 -> Sum3/1
  Mux3/1 -> Demux3/1

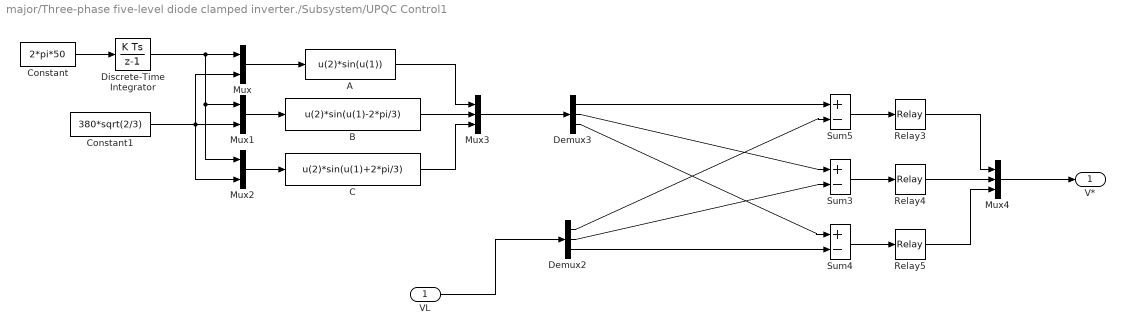
== system major/Three-phase five-level diode clamped inverter./Subsystem/UPQC Control1 ==
  VL : Inport
  A : Fcn  Expr=u(2)*sin(u(1))
  B : Fcn  Expr=u(2)*sin(u(1)-2*pi/3)
  C : Fcn  Expr=u(2)*sin(u(1)+2*pi/3)
  Constant : Constant  Value=2*pi*50  OutDataType=fixdt(1, 16)  OutScaling=2^0
  Constant1 : Constant  Value=380*sqrt(2/3)  OutDataType=fixdt(1, 16)  OutScaling=2^0
  Demux2 : Demux  Outputs=3
  Demux3 : Demux  Outputs=3
  Discrete-Time Integrator : DiscreteIntegrator  SampleTime=Ts  OutDataType=fixdt(1, 16)  OutScaling=2^0  ICPrevOutput=DiscIntNeverNeededParam  ICPrevScaledInput=DiscIntNeverNeededParam
  Mux : Mux  Inputs=2
  Mux1 : Mux  Inputs=2
  Mux2 : Mux  Inputs=2
  Mux3 : Mux  Inputs=3
  Mux4 : Mux  Inputs=3
  Relay3 : Relay  OnSwitchValue=1  OffSwitchValue=-1  OutDataType=fixdt(1, 16)  OutScaling=2^0
  Relay4 : Relay  OnSwitchValue=1  OffSwitchValue=-1  OutDataType=fixdt(1, 16)  OutScaling=2^0
  Relay5 : Relay  OnSwitchValue=1  OffSwitchValue=-1  OutDataType=fixdt(1, 16)  OutScaling=2^0
  Sum3 : Sum  Inputs=+-  OutDataType=fixdt(1, 16)  OutScaling=2^0
  Sum4 : Sum  Inputs=+-  OutDataType=fixdt(1, 16)  OutScaling=2^0
  Sum5 : Sum  Inputs=+-  OutDataType=fixdt(1, 16)  OutScaling=2^0
  V* : Outport  OutDataType=fixdt(1, 16)  OutScaling=2^0
  wires:
  Constant/1 -> Discrete-Time Integrator/1
  Discrete-Time Integrator/1 -> Mux/1, Mux2/1, Mux1/1
  Constant1/1 -> Mux/2, Mux1/2, Mux2/2
  Mux/1 -> A/1
  Mux1/1 -> B/1
  Mux2/1 -> C/1
  A/1 -> Mux3/1
  B/1 -> Mux3/2
  C/1 -> Mux3/3
  Sum5/1 -> Relay3/1
  Sum3/1 -> Relay4/1
  Sum4/1 -> Relay5/1
  Relay3/1 -> Mux4/1
  Relay4/1 -> Mux4/2
  Relay5/1 -> Mux4/3
  Mux4/1 -> V*/1
  VL/1 -> Demux2/1
  Demux3/1 -> Sum5/1
  Demux2/3 -> Sum4/2
  Demux2/1 -> Sum5/2
  Demux3/3 -> Sum4/1
  Demux2/2 -> Sum3/2
  Demux3/2 -> Sum3/1
  Mux3/1 -> Demux3/1

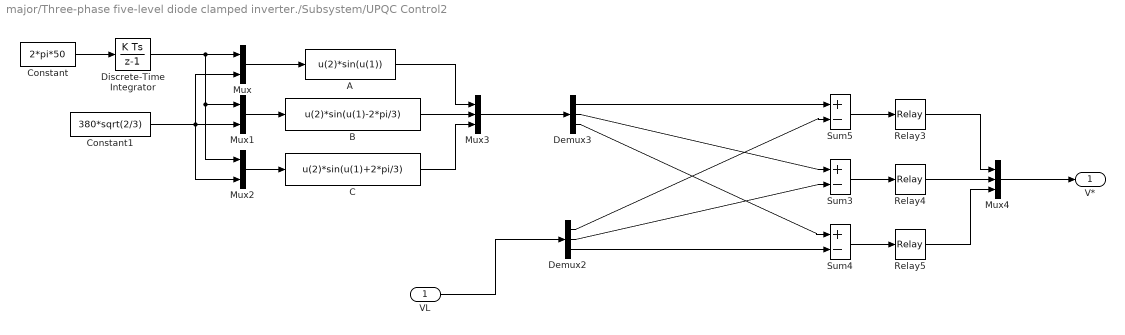
== system major/Three-phase five-level diode clamped inverter./Subsystem/UPQC Control2 ==
  VL : Inport
  A : Fcn  Expr=u(2)*sin(u(1))
  B : Fcn  Expr=u(2)*sin(u(1)-2*pi/3)
  C : Fcn  Expr=u(2)*sin(u(1)+2*pi/3)
  Constant : Constant  Value=2*pi*50  OutDataType=fixdt(1, 16)  OutScaling=2^0
  Constant1 : Constant  Value=380*sqrt(2/3)  OutDataType=fixdt(1, 16)  OutScaling=2^0
  Demux2 : Demux  Outputs=3
  Demux3 : Demux  Outputs=3
  Discrete-Time Integrator : DiscreteIntegrator  SampleTime=Ts  OutDataType=fixdt(1, 16)  OutScaling=2^0  ICPrevOutput=DiscIntNeverNeededParam  ICPrevScaledInput=DiscIntNeverNeededParam
  Mux : Mux  Inputs=2
  Mux1 : Mux  Inputs=2
  Mux2 : Mux  Inputs=2
  Mux3 : Mux  Inputs=3
  Mux4 : Mux  Inputs=3
  Relay3 : Relay  OnSwitchValue=1  OffSwitchValue=-1  OutDataType=fixdt(1, 16)  OutScaling=2^0
  Relay4 : Relay  OnSwitchValue=1  OffSwitchValue=-1  OutDataType=fixdt(1, 16)  OutScaling=2^0
  Relay5 : Relay  OnSwitchValue=1  OffSwitchValue=-1  OutDataType=fixdt(1, 16)  OutScaling=2^0
  Sum3 : Sum  Inputs=+-  OutDataType=fixdt(1, 16)  OutScaling=2^0
  Sum4 : Sum  Inputs=+-  OutDataType=fixdt(1, 16)  OutScaling=2^0
  Sum5 : Sum  Inputs=+-  OutDataType=fixdt(1, 16)  OutScaling=2^0
  V* : Outport  OutDataType=fixdt(1, 16)  OutScaling=2^0
  wires:
  Constant/1 -> Discrete-Time Integrator/1
  Discrete-Time Integrator/1 -> Mux/1, Mux2/1, Mux1/1
  Constant1/1 -> Mux/2, Mux1/2, Mux2/2
  Mux/1 -> A/1
  Mux1/1 -> B/1
  Mux2/1 -> C/1
  A/1 -> Mux3/1
  B/1 -> Mux3/2
  C/1 -> Mux3/3
  Sum5/1 -> Relay3/1
  Sum3/1 -> Relay4/1
  Sum4/1 -> Relay5/1
  Relay3/1 -> Mux4/1
  Relay4/1 -> Mux4/2
  Relay5/1 -> Mux4/3
  Mux4/1 -> V*/1
  VL/1 -> Demux2/1
  Demux3/1 -> Sum5/1
  Demux2/3 -> Sum4/2
  Demux2/1 -> Sum5/2
  Demux3/3 -> Sum4/1
  Demux2/2 -> Sum3/2
  Demux3/2 -> Sum3/1
  Mux3/1 -> Demux3/1
